simulink model "two_dof_arm_dynamics"  (R2023a)
settings: Solver=FixedStepAuto  StartTime=0.0  StopTime=1  FixedStep=0.001  RelTol=1e-3
InitFcn:
  | m1 = 2;
  | m2 = 1;
  | l1 = 2;
  | l2 = 1;
  | g = -9.81;
settings Model: Creator=Jordan  LastModifiedBy=jorda
settings OptimizationCC: ReuseModelBlockBuffer=off

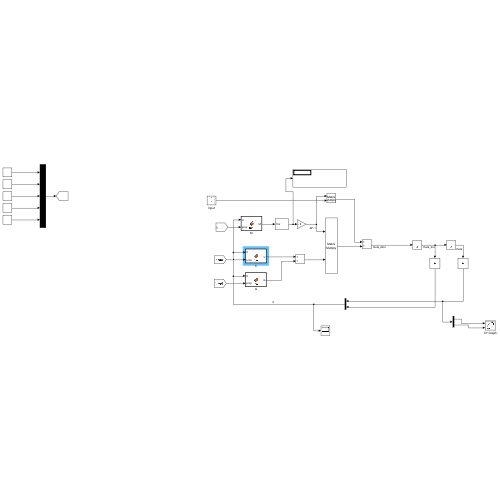
[thumbnail: Simulink's stored preview of the top-level diagram]
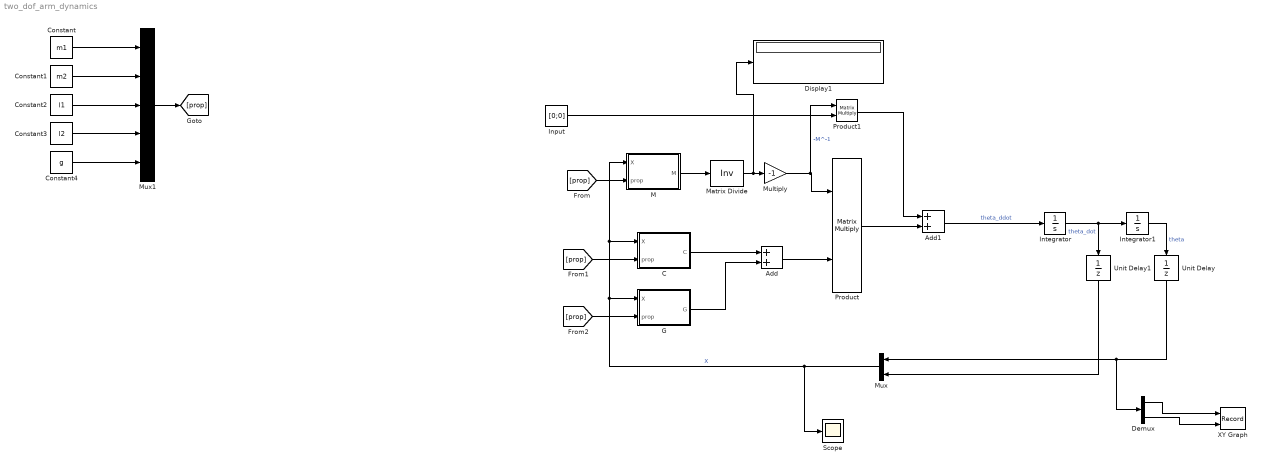
== system two_dof_arm_dynamics ==
  Add : Sum
  Add1 : Sum
  C : MATLAB Function  TreatAsAtomicUnit=on
  Constant : Constant  Value=m1
  Constant1 : Constant  Value=m2
  Constant2 : Constant  Value=l1
  Constant3 : Constant  Value=l2
  Constant4 : Constant  Value=g
  Demux : Demux  Outputs=2
  Display1 : Display
  G : MATLAB Function  TreatAsAtomicUnit=on
  Input : Constant  Value=[0;0]  VectorParams1D=off
  Integrator : Integrator  InitialCondition=[0;0]  ContinuousStateAttributes='velocity'
  Integrator1 : Integrator  InitialCondition=[pi/4;0]  ContinuousStateAttributes='position'
  M : MATLAB Function  TreatAsAtomicUnit=on
  Matrix Divide : Product  Inputs=/  Multiplication=Matrix(*)
  Multiply : Gain  Gain=-1
  Mux : Mux  Inputs=2
  Mux1 : Mux  Inputs=5
  Product : Product  Multiplication=Matrix(*)
  Product1 : Product  Multiplication=Matrix(*)
  Scope : Scope
  Unit Delay : UnitDelay  InitialCondition=[0;0]  SampleTime=-1  HasFrameUpgradeWarning=on
  Unit Delay1 : UnitDelay  InitialCondition=[0;0]  SampleTime=-1  HasFrameUpgradeWarning=on
  XY Graph : Record  FileSettingsInternal="{\"entries\":[{\"content\":{\"excelSettings\":{\"content\":{},\"type\":\"Streamout.ExcelSettings\"}},\"type\":\"Streamout.FileSettingStorage\",\"uuid\":\"db7e0583-9c7d-4443-9480-6a2a406ff6bf\"}],\"packageUris\":[\"http://schema.mathworks.com/mf0/streamout_blocks/R2020a\"],\"version\":\"1.0\"}"  Layout=[1 1]  SignalsInternal="{\"entries\":[{\"content\":{\"signals\":[{\"content\":{\"blockPath\":[\"two_dof_arm_dynamics/XY Graph\"],\"dimensions\":[1,1],\"domain\":\"two_dof_arm_dynamics/XY Graph\",\"lineColor\":\"#a2142f\",\"plots\":[1],\"port\":1,\"signalID\":8,\"signalName\":\"Demux:1\"},\"type\":\"RecordBlkView.Signal\",\"uuid\":\"d5333efc-7c0c-4144-8aea-124f5ad81557\"},{\"content\":{\"blockPath\":[\"two_dof_arm_dynamics/XY Graph\"],\"dimensions\":[1,1],\"domain\":\"two_dof_arm_dynamics/XY Graph\",\"lineColor\":\"#139fff\",\"plots\":[1],\"port\":2,\"signalID\":11,\"signalName\":\"Demux:2\"},\"type\":\"RecordBlkView.Signal\",\"uuid\":\"e6d19277-b0eb-4834-adfe-c9bdf2a13e94\"}]},\"type\":\"RecordBlkView.InputSignals\",\"uuid\":\"2fae9b3a-1bb7-450d-9554-a8b7e6070ae3\"}],\"packageUris\":[\"http://schema.mathworks.com/mf0/streamout_blocks/R2020a\"],\"version\":\"1.0\"}"  VisualizationBindings="{\"xyplotplugin\":{\"info\":[{\"series\":[{\"bindingParametersList\":[{\"parameter\":\"X-Axis\",\"signalID\":8,\"signalName\":\"Demux:1\"},{\"parameter\":\"Y-Axis\",\"signalID\":11,\"signalName\":\"Demux:2\"}],\"seriesID\":13228}],\"subplotID\":1}]}}"  CompatibilityTag=XY
  wires:
  M/1(M) -> Matrix Divide/1
  Matrix Divide/1 -> Display1/1, Multiply/1
  Multiply/1 -> Product1/1, Product/1  "-M^-1"
  Add/1 -> Product/2
  C/1(C) -> Add/1
  G/1(G) -> Add/2
  Product/1 -> Add1/2
  Product1/1 -> Add1/1
  Add1/1 -> Integrator/1  "theta_ddot"
  Integrator/1 -> Unit Delay1/1, Integrator1/1  "theta_dot"
  Integrator1/1 -> Unit Delay/1  "theta"
  Mux/1 -> Scope/1, G/1(X), C/1(X), M/1(X)  "X"
  Constant/1 -> Mux1/1
  Constant1/1 -> Mux1/2
  Constant2/1 -> Mux1/3
  Constant3/1 -> Mux1/4
  Constant4/1 -> Mux1/5
  Mux1/1 -> [prop]
  [prop] -> M/2(prop)
  [prop] -> C/2(prop)
  [prop] -> G/2(prop)
  Input/1 -> Product1/2
  Unit Delay/1 -> Demux/1, Mux/1
  Unit Delay1/1 -> Mux/2
  Demux/1 -> XY Graph/1
  Demux/2 -> XY Graph/2

== matlab function two_dof_arm_dynamics/M ==
  data: X input; M output; prop input
function M = fcn(X,prop)
    m1 = prop(1);
    m2 = prop(2);
    l1 = prop(3);
    l2 = prop(4);
    r1 = l1/2;
    r2 = l2/2;
    theta1 = X(1);
    theta2 = X(2);
    Iz1 = 1/12*m1*l1^2;
    Iz2 = 1/12*m2*l2^2;
    
    M11 = m2*l1^2+2*m2cos(theta2)*l1*(l2/2)+m1*r1^2+m2*r2^2+Iz1+Iz2;
    M12 = m2*r2^2+l1*m2*cos(theta2)*r2+Iz2;
    M21 = m2*r2^2+l1*m2*cos(theta2)*r2+Iz2;
    M22 = m2*r2^2+Iz2;
    
    M = [M11 M12; M21 M22];

== matlab function two_dof_arm_dynamics/G ==
  data: X input; G output; prop input
function G = fcn(X,prop)
    m1 = prop(1);
    m2 = prop(2);
    l1 = prop(3);
    l2 = prop(4);
    g = prop(5);
    theta1 = X(1);
    theta2 = X(2);
    r1 = l1/2;
    r2 = l2/2;
    eta = m2*l1*l2;
    alpha = (m1+m2)*l1^2;
    epsilon = g*l2;
    
    G1 = g*m2*(r2*cos(q1+q2)+l1*cos(theta1))+g*m1*r1*cos(theta1);
    G2 = g*m2*r2*cos(theta1+theta2);
    
    G = [G1;G2];

== matlab function two_dof_arm_dynamics/C ==
  data: X input; C output; prop input
function C = fcn(X,prop)
    m2 = prop(2);
    l1 = prop(3);
    l2 = prop(4);
    r2 = l2/2;
    theta1 = X(1);
    theta2 = X(2);
    theta1_dot = X(3);
    theta2_dot = X(4);
    eta = m2*l1*l2;
    
    V11 = -l1*m2*theta2_dot*sin(theta2);
    V12 = -l1*m2*r2*sin(theta2)*(theta1_dot+theta2_dot);
    V21 = l1*m2*theta1_dot*r2*sin(theta2);
    V22 = 0
    
    C = [V11 V12;V21 V22];
